simulink model "formula_0508a"  (R2019a)
settings: Solver=VariableStepAuto  StartTime=0.0  StopTime=10.0  RelTol=1e-3
values from neighbouring files (symbols this model uses):
  a0 = 1.3    [mf.mat]    (also in model_2r.m; model_Fy.m)
  a1 = -0.0274    [mf.mat]    (also in model_2r.m; model_Fy.m)
  a10 = 0.015    [mf.mat]    (also in model_2r.m; model_Fy.m)
  a11 = 0.00849    [mf.mat]    (also in model_2r.m = 0.0849; model_Fy.m)
  a12 = -0.0103    [mf.mat]    (also in model_2r.m; model_Fy.m)
  a13 = 0.0395    [mf.mat]    (also in model_2r.m; model_Fy.m)
  a2 = 1.05    [mf.mat]    (also in model_2r.m; model_Fy.m)
  a3 = 1.18    [mf.mat]    (also in model_2r.m; model_Fy.m)
  a4 = 7.69    [mf.mat]    (also in model_2r.m; model_Fy.m)
  a5 = 0.009    [mf.mat]    (also in model_2r.m; model_Fy.m)
  a6 = -0.257    [mf.mat]    (also in model_2r.m; model_Fy.m)
  a7 = 0.224    [mf.mat]    (also in model_2r.m; model_Fy.m)
  a8 = 0.025    [mf.mat]    (also in model_2r.m; model_Fy.m)
  a9 = 0.01    [mf.mat]    (also in model_2r.m; model_Fy.m)
settings Model: Creator=Shingo Haketa  LastModifiedBy=Shingo Haketa

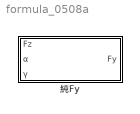
== system formula_0508a ==
  純Fy : Subsystem

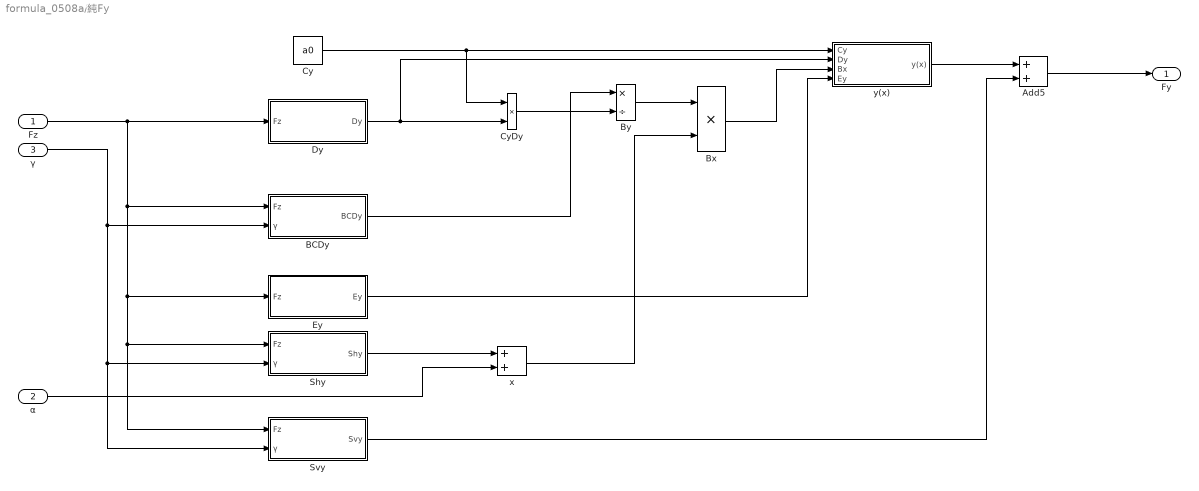
== system formula_0508a/純Fy ==
  Fz : Inport
  α : Inport  Port=2
  γ : Inport  Port=3
  Add5 : Sum
  BCDy : Subsystem
  Bx : Product
  By : Product  Inputs=*/
  Cy : Constant  Value=a0
  CyDy : Product
  Dy : Subsystem
  Ey : Subsystem
  Shy : Subsystem
  Svy : Subsystem
  x : Sum
  y(x) : Subsystem
  Fy : Outport  VectorParamsAs1DForOutWhenUnconnected=off
  wires:
  Ey/1(Ey) -> y(x)/4(Ey)
  γ/1 -> Svy/2(γ), Shy/2(γ), BCDy/2(γ)
  y(x)/1(y(x)) -> Add5/1
  Fz/1 -> Dy/1(Fz), Svy/1(Fz), Shy/1(Fz), Ey/1(Fz), BCDy/1(Fz)
  Svy/1(Svy) -> Add5/2
  Cy/1 -> CyDy/1, y(x)/1(Cy)
  CyDy/1 -> By/2
  Dy/1(Dy) -> CyDy/2, y(x)/2(Dy)
  Add5/1 -> Fy/1
  By/1 -> Bx/1
  BCDy/1(BCDy) -> By/1
  α/1 -> x/2
  Shy/1(Shy) -> x/1
  x/1 -> Bx/2
  Bx/1 -> y(x)/3(Bx)

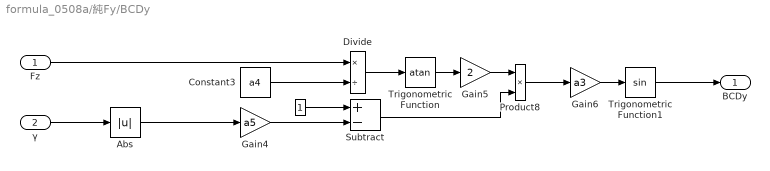
== system formula_0508a/純Fy/BCDy ==
  Fz : Inport
  γ : Inport  Port=2
  " " : Constant
  Abs : Abs
  Constant3 : Constant  Value=a4
  Divide : Product  Inputs=*/
  Gain4 : Gain  Gain=a5
  Gain5 : Gain  Gain=2
  Gain6 : Gain  Gain=a3
  Product8 : Product
  Subtract : Sum  Inputs=+-
  Trigonometric Function : Trigonometry  Operator=atan
  Trigonometric Function1 : Trigonometry
  BCDy : Outport
  wires:
  Gain6/1 -> Trigonometric Function1/1
  Divide/1 -> Trigonometric Function/1
  Gain4/1 -> Subtract/2
  Product8/1 -> Gain6/1
  Subtract/1 -> Product8/2
  γ/1 -> Abs/1
  Abs/1 -> Gain4/1
  Trigonometric Function/1 -> Gain5/1
  Gain5/1 -> Product8/1
  " "/1 -> Subtract/1
  Fz/1 -> Divide/1
  Constant3/1 -> Divide/2
  Trigonometric Function1/1 -> BCDy/1

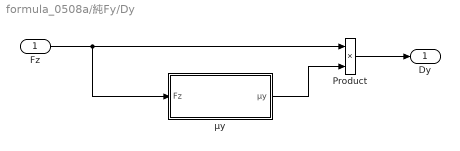
== system formula_0508a/純Fy/Dy ==
  Fz : Inport
  Product : Product
  μy : Subsystem
  Dy : Outport
  wires:
  μy/1(μy) -> Product/2
  Fz/1 -> μy/1(Fz), Product/1
  Product/1 -> Dy/1

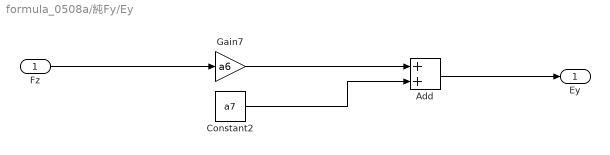
== system formula_0508a/純Fy/Ey ==
  Fz : Inport
  Add : Sum
  Constant2 : Constant  Value=a7
  Gain7 : Gain  Gain=a6
  Ey : Outport
  wires:
  Gain7/1 -> Add/1
  Constant2/1 -> Add/2
  Fz/1 -> Gain7/1
  Add/1 -> Ey/1

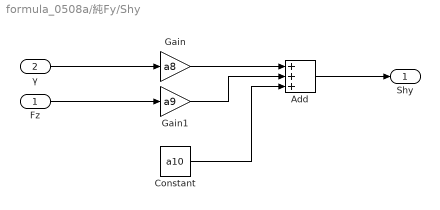
== system formula_0508a/純Fy/Shy ==
  Fz : Inport
  γ : Inport  Port=2
  Add : Sum  Inputs=+++
  Constant : Constant  Value=a10
  Gain : Gain  Gain=a8
  Gain1 : Gain  Gain=a9
  Shy : Outport
  wires:
  Gain1/1 -> Add/2
  Constant/1 -> Add/3
  Fz/1 -> Gain1/1
  γ/1 -> Gain/1
  Gain/1 -> Add/1
  Add/1 -> Shy/1

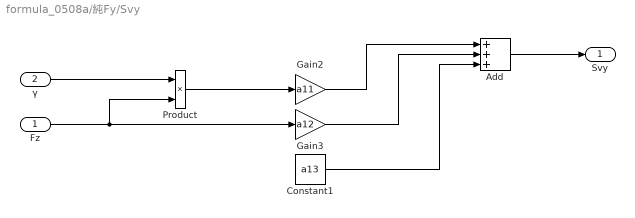
== system formula_0508a/純Fy/Svy ==
  Fz : Inport
  γ : Inport  Port=2
  Add : Sum  Inputs=+++
  Constant1 : Constant  Value=a13
  Gain2 : Gain  Gain=a11
  Gain3 : Gain  Gain=a12
  Product : Product
  Svy : Outport
  wires:
  Gain2/1 -> Add/1
  Product/1 -> Gain2/1
  Gain3/1 -> Add/2
  Fz/1 -> Product/2, Gain3/1
  Constant1/1 -> Add/3
  γ/1 -> Product/1
  Add/1 -> Svy/1

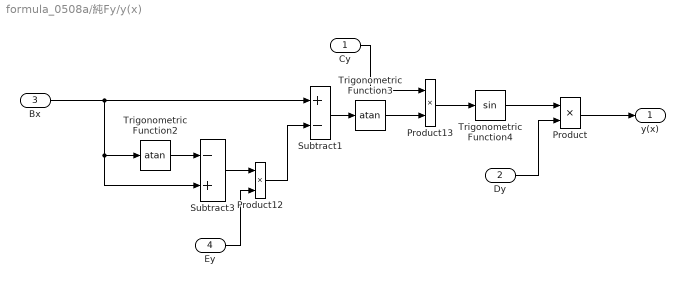
== system formula_0508a/純Fy/y(x) ==
  Cy : Inport
  Dy : Inport  Port=2
  Bx : Inport  Port=3
  Ey : Inport  Port=4
  Product : Product
  Product12 : Product
  Product13 : Product
  Subtract1 : Sum  Inputs=+-
  Subtract3 : Sum  Inputs=-+
  Trigonometric Function2 : Trigonometry  Operator=atan
  Trigonometric Function3 : Trigonometry  Operator=atan
  Trigonometric Function4 : Trigonometry
  y(x) : Outport
  wires:
  Dy/1 -> Product/2
  Subtract3/1 -> Product12/1
  Product13/1 -> Trigonometric Function4/1
  Product12/1 -> Subtract1/2
  Trigonometric Function2/1 -> Subtract3/1
  Subtract1/1 -> Trigonometric Function3/1
  Trigonometric Function3/1 -> Product13/2
  Product/1 -> y(x)/1
  Bx/1 -> Subtract3/2, Trigonometric Function2/1, Subtract1/1
  Cy/1 -> Product13/1
  Ey/1 -> Product12/2
  Trigonometric Function4/1 -> Product/1

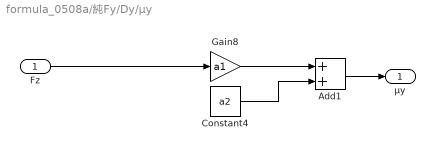
== system formula_0508a/純Fy/Dy/μy ==
  Fz : Inport
  Add1 : Sum
  Constant4 : Constant  Value=a2
  Gain8 : Gain  Gain=a1
  μy : Outport
  wires:
  Fz/1 -> Gain8/1
  Gain8/1 -> Add1/1
  Add1/1 -> μy/1
  Constant4/1 -> Add1/2
